simulink model "MotionPlanner"  (R2024b)
settings: Solver=FixedStepAuto  StartTime=0.0  StopTime=10.0  MaxStep=0.02  RelTol=1e-3  EnableMultiTasking=on
undefined symbols (not defined in the file or in its folder): actorProfiles, computeMethod, replanRate, timeResolution, Ts
libraries: simulink x1
settings Model: Creator=The MathWorks, Inc.  LastModifiedBy=The MathWorks, Inc.
settings SolverCC: AlgebraicLoopSolver=TrustRegion  MaxZcPerStep=1
settings OptimizationCC: DefaultParameterBehavior=Inlined  InlineInvariantSignals=on  EnhancedBackFolding=on  PassReuseOutputArgsAs=Individual arguments  ZeroExternalMemoryAtStartup=off  ZeroInternalMemoryAtStartup=off  EfficientFloat2IntCast=on  OptimizeBlockOrder=speed  DifferentSizesBufferReuse=on  OptimizationCustomize=off  EfficientTunableParamExpr=on
settings DebuggingCC: ParameterTunabilityLossMsg=error  UnconnectedInputMsg=warning  UnconnectedOutputMsg=warning  UnconnectedLineMsg=warning  ModelReferenceSymbolNameMessage=none  SubsystemReferenceDiagnosticForUnitTest=warning
settings HardwareCC: ProdLongLongMode=on
settings ModelReferenceCC: EnableRefExpFcnMdlSchedulingChecks=on  PropagateVarSize=During execution
settings RTWCC: Description=Embedded Coder  SystemTargetFile=ert.tlc  TemplateMakefile=ert_default_tmf  RTWVerbose=off  BuildConfiguration=Faster Runs  PortableWordSizes=on  TargetLang=C++  GPUComputeCapability=3.5  DLArmComputeVersion=19.05
settings CodeAppCC: ForceParamTrailComments=on  IgnoreCustomStorageClasses=off  OperatorAnnotations=on  SimulinkDataObjDesc=on  SFDataObjDesc=on  CustomSymbolStrGlobalVar=$N$M  CustomSymbolStrType=$N$M_T  CustomSymbolStrFcn=APV_$N$M$F  CustomSymbolStrMacro=$N$M  InsertBlockDesc=on
settings ERTTargetCC: TargetLangStandard=C++03 (ISO)  GenerateSampleERTMain=on  CombineSignalStateStructs=on  CodeInterfacePackaging=C++ class  SupportVariableSizeSignals=on  RootIOFormat=Structure reference  ERTCustomFileTemplate=example_file_process.tlc  DynamicArrayContainerType=coder::array

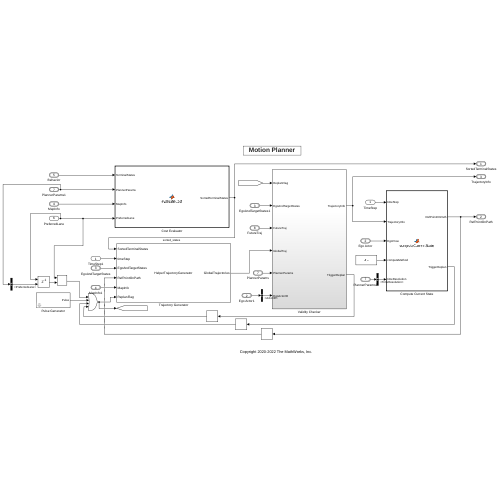
[thumbnail: Simulink's stored preview of the top-level diagram]
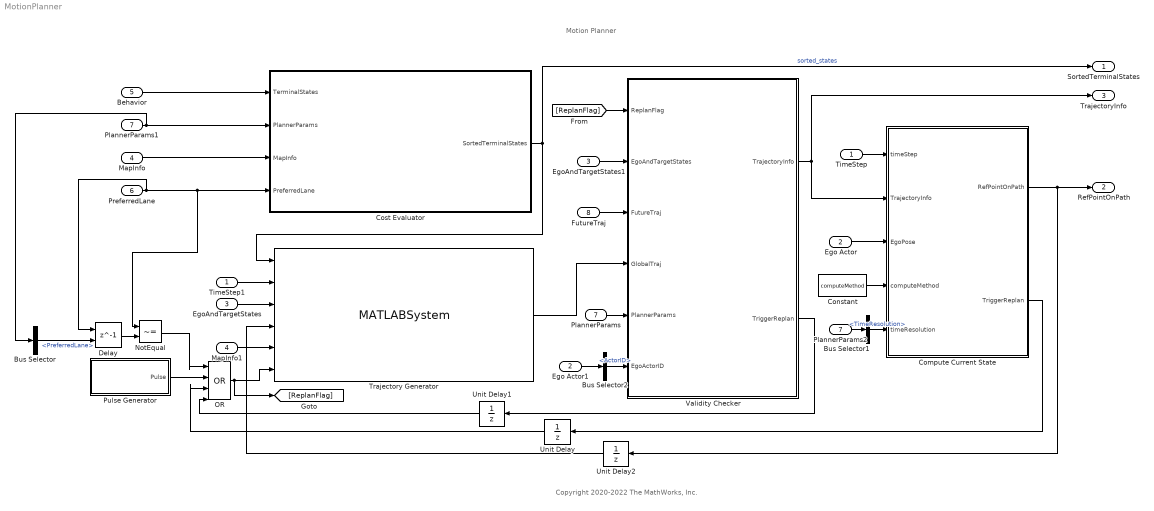
== system MotionPlanner ==
  note: Motion Planner
  note: Copyright 2020-2022 The MathWorks, Inc.
  TimeStep : Inport
  Ego Actor : Inport  Port=2  OutDataTypeStr=Bus: BusVehiclePose  Unit=m  BusOutputAsStruct=on
  EgoAndTargetStates : Inport  Port=3  OutDataTypeStr=Bus: BusEgoAndTargetStates  BusOutputAsStruct=on
  MapInfo : Inport  Port=4  OutDataTypeStr=Bus: BusMapInfo  BusOutputAsStruct=on
  Behavior : Inport  Port=5  OutDataTypeStr=Bus: BusTerminalStatesCombinations
  PreferredLane : Inport  Port=6
  PlannerParams : Inport  Port=7  OutDataTypeStr=Bus: BusPlannerParams  BusOutputAsStruct=on
  FutureTraj : Inport  Port=8  OutDataTypeStr=Bus: BusPredictedTrajectories  BusOutputAsStruct=on
  Bus Selector : BusSelector  OutputSignals=PreferredLane
  Bus Selector1 : BusSelector  OutputSignals=TimeResolution
  Bus Selector2 : BusSelector  OutputSignals=ActorID
  Compute Current State : MATLAB Function  TreatAsAtomicUnit=on
  Constant : Constant  Value=computeMethod
  Cost Evaluator : MATLAB Function  TreatAsAtomicUnit=on
  Delay : Delay  DelayLength=1  InitialConditionSource=Input port
      settings: InputPortMap=u0,p4
  Ego Actor1 : InportShadow  Port=2  OutDataTypeStr=Bus: BusVehiclePose  Unit=m  BusOutputAsStruct=on
  EgoAndTargetStates1 : InportShadow  Port=3  OutDataTypeStr=Bus: BusEgoAndTargetStates  BusOutputAsStruct=on
  MapInfo1 : InportShadow  Port=4  OutDataTypeStr=Bus: BusMapInfo  BusOutputAsStruct=on
  NotEqual : RelationalOperator  Operator=~=  OutDataTypeStr=boolean  RndMeth=Simplest  InputSameDT=off
  OR : Logic  Operator=OR  Inputs=4  IconShape=distinctive  AllPortsSameDT=off  OutDataTypeStr=boolean
  PlannerParams1 : InportShadow  Port=7  OutDataTypeStr=Bus: BusPlannerParams  BusOutputAsStruct=on
  PlannerParams2 : InportShadow  Port=7  OutDataTypeStr=Bus: BusPlannerParams  BusOutputAsStruct=on
  Pulse Generator : Subsystem  mask(Pulse Generator){pulsePeriod=1/replanRate, sampleTime=timeResolution}
      mask prompts: pulsePeriod "Pulse period (sec)"; sampleTime "Sample time (sec)"
      mask help: Generates a periodic pulse. The pulse is high for the first sample of the period and then is low for the remained of the period.
  TimeStep1 : InportShadow
  Trajectory Generator : MATLABSystem  System=HelperTrajectoryGenerator  SimulateUsing=Interpreted execution
      mask Type: HelperTrajectoryGenerator
      mask Display:
      | disp('HelperTrajectoryGenerator');
      | port_label('input',1,'SortedTerminalStates');
      | port_label('input',2,'timeStep');
      | port_label('input',3,'EgoAndTargetStates');
      | port_label('input',4,'RefPointOnPath');
      | port_label('input',5,'MapInfo');
      | port_label('input',6,'ReplanFlag');
      | port_label('output',1,'GlobalTrajectories');
  Unit Delay : UnitDelay  InitialCondition=false  SampleTime=-1  HasFrameUpgradeWarning=on
  Unit Delay1 : UnitDelay  InitialCondition=false  SampleTime=-1  HasFrameUpgradeWarning=on
  Unit Delay2 : UnitDelay  SampleTime=-1  HasFrameUpgradeWarning=on
  Validity Checker : Subsystem
  SortedTerminalStates : Outport  OutDataTypeStr=Bus: BusTerminalStatesCombinations  BusOutputAsStruct=on
  RefPointOnPath : Outport  Port=2  OutDataTypeStr=Bus: BusRefPointOnPath
  TrajectoryInfo : Outport  Port=3  OutDataTypeStr=Bus: BusGlobalTrajectories  BusOutputAsStruct=on
  wires:
  NotEqual/1 -> OR/1
  PlannerParams1/1 -> Bus Selector/1, Cost Evaluator/2(PlannerParams)
  PreferredLane/1 -> NotEqual/1, Cost Evaluator/4(PreferredLane), Delay/1
  Unit Delay1/1 -> OR/4
  Compute Current State/1(RefPointOnPath) -> RefPointOnPath/1, Unit Delay2/1
  Ego Actor/1 -> Compute Current State/3(EgoPose)
  Cost Evaluator/1(SortedTerminalStates) -> SortedTerminalStates/1, Trajectory Generator/1  "sorted_states"
  [ReplanFlag] -> Validity Checker/1(ReplanFlag)
  Ego Actor1/1 -> Bus Selector2/1
  Delay/1 -> NotEqual/2
  MapInfo/1 -> Cost Evaluator/3(MapInfo)
  TimeStep1/1 -> Trajectory Generator/2
  Constant/1 -> Compute Current State/4(computeMethod)
  Bus Selector1/1 -> Compute Current State/5(timeResolution)  "<TimeResolution>"
  TimeStep/1 -> Compute Current State/1(timeStep)
  PlannerParams2/1 -> Bus Selector1/1
  Pulse Generator/1(Pulse) -> OR/2
  Bus Selector2/1 -> Validity Checker/6(EgoActorID)  "<ActorID>"
  Compute Current State/2(TriggerReplan) -> Unit Delay/1
  MapInfo1/1 -> Trajectory Generator/5
  Bus Selector/1 -> Delay/2  "<PreferredLane>"
  Unit Delay2/1 -> Trajectory Generator/4
  OR/1 -> Trajectory Generator/6, [ReplanFlag]
  Unit Delay/1 -> OR/3
  Validity Checker/2(TriggerReplan) -> Unit Delay1/1
  FutureTraj/1 -> Validity Checker/3(FutureTraj)
  Behavior/1 -> Cost Evaluator/1(TerminalStates)
  EgoAndTargetStates/1 -> Trajectory Generator/3
  Validity Checker/1(TrajectoryInfo) -> Compute Current State/2(TrajectoryInfo), TrajectoryInfo/1
  EgoAndTargetStates1/1 -> Validity Checker/2(EgoAndTargetStates)
  PlannerParams/1 -> Validity Checker/5(PlannerParams)
  Trajectory Generator/1 -> Validity Checker/4(GlobalTraj)

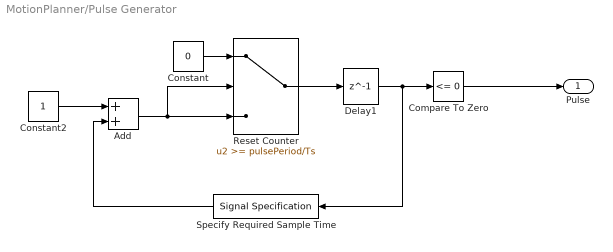
== system MotionPlanner/Pulse Generator ==
  Add : Sum
  Compare To Zero : simulink/Logic and Bit Operations/Compare To Zero  relop=<=  OutDataTypeStr=boolean
  Constant : Constant  Value=0
  Constant2 : Constant
  Delay1 : Delay  DelayLength=1
  Reset Counter : Switch  Threshold=pulsePeriod/Ts  SaturateOnIntegerOverflow=off  InputSameDT=off
      settings: AttributesFormatString=|
      | ----------------------------
      | Threshold = %<Threshold>
  Specify Required Sample Time : SignalSpecification  SampleTime=sampleTime
  Pulse : Outport
  wires:
  Reset Counter/1 -> Delay1/1
  Add/1 -> Reset Counter/3, Reset Counter/2
  Specify Required Sample Time/1 -> Add/2
  Delay1/1 -> Specify Required Sample Time/1, Compare To Zero/1
  Constant2/1 -> Add/1
  Constant/1 -> Reset Counter/1
  Compare To Zero/1 -> Pulse/1

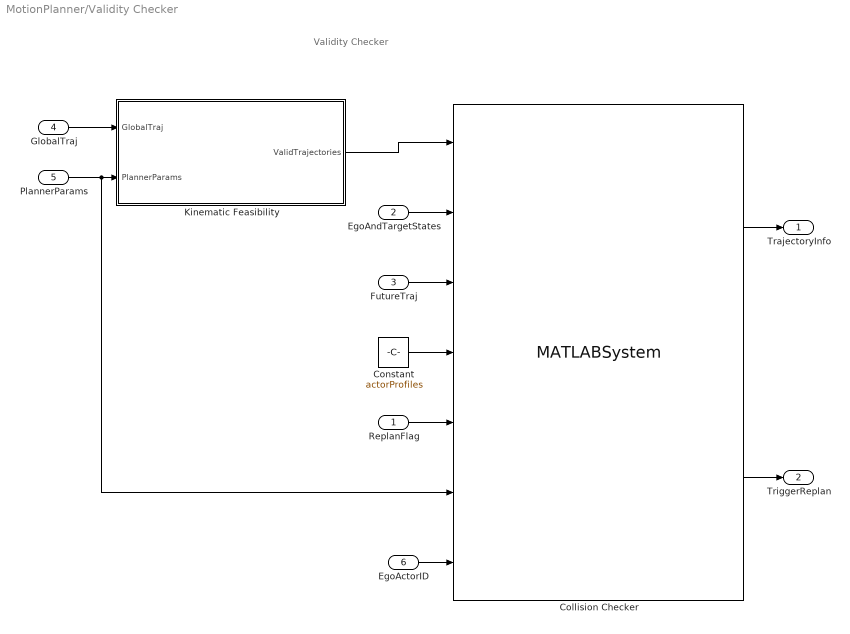
== system MotionPlanner/Validity Checker ==
  note: Validity Checker
  ReplanFlag : Inport
  EgoAndTargetStates : Inport  Port=2
  FutureTraj : Inport  Port=3
  GlobalTraj : Inport  Port=4
  PlannerParams : Inport  Port=5  OutDataTypeStr=Bus: BusPlannerParams
  EgoActorID : Inport  Port=6
  Collision Checker : MATLABSystem  System=HelperCollisionChecker  SimulateUsing=Interpreted execution
      mask Type: HelperCollisionChecker
      mask Display:
      | disp('HelperCollisionChecker');
      | port_label('input',1,'ValidTrajectories');
      | port_label('input',2,'EgoAndTargetStates');
      | port_label('input',3,'FutureTrajectory');
      | port_label('input',4,'VehicleProfiles');
      | port_label('input',5,'ReplanFlag');
      | port_label('input',6,'PlannerParams');
      | port_label('input',7,'EgoID');
      | port_label('output',1,'TrajectoryInfo');
      | port_label('output',2,'TriggerReplan');
  Constant : Constant  Value=actorProfiles  OutDataTypeStr=Bus: BusActorProfiles
  Kinematic Feasibility : MATLAB Function  TreatAsAtomicUnit=on
  TrajectoryInfo : Outport
  TriggerReplan : Outport  Port=2
  wires:
  Collision Checker/1 -> TrajectoryInfo/1
  FutureTraj/1 -> Collision Checker/3
  ReplanFlag/1 -> Collision Checker/5
  Constant/1 -> Collision Checker/4
  Kinematic Feasibility/1(ValidTrajectories) -> Collision Checker/1
  EgoAndTargetStates/1 -> Collision Checker/2
  Collision Checker/2 -> TriggerReplan/1
  GlobalTraj/1 -> Kinematic Feasibility/1(GlobalTraj)
  PlannerParams/1 -> Collision Checker/6, Kinematic Feasibility/2(PlannerParams)
  EgoActorID/1 -> Collision Checker/7

== matlab function MotionPlanner/Compute Current State ==
  data: timeStep input; TrajectoryInfo input; RefPointOnPath output Bus: BusRefPointOnPath; EgoPose input; TriggerReplan output; computeMethod input; timeResolution input
function [RefPointOnPath, TriggerReplan]  = computeCurrentState(timeStep, TrajectoryInfo,...
                                            EgoPose, computeMethod, timeResolution)...
%computeCurrentState estimates the next state of the vehicle based on the
%time or current pose of the ego vehicle.
%
% This function block estimate sthe current pose of the ego vehicle based
% on time or based on current ego pose based on the input from
% StateSelector. If the StateSelector is zero it estimates the pose based
% on current pose, otherwise it estimates state based on time.

persistent replanTime refPosePrev refCurvPrev refVelPrev refAccPrev sectionStartIndexPrev time
if isempty(replanTime)
    replanTime = 0;
    refPosePrev = zeros(1,3);
    refCurvPrev = 0;
    refVelPrev = 0;
    refAccPrev = 0;
    sectionStartIndexPrev = 0;
    time = 0;
end

if TrajectoryInfo.IsNew
    replanTime = time;
end

% Initialize output structure
RefPointOnPath = HelperLCPlannerDefaultData.RefPointOnPath;

optimalTrajIndex = TrajectoryInfo.OptimalTrajectoryIndex;
optimalTrajectory = TrajectoryInfo.GlobalTrajectory(optimalTrajIndex).Trajectory;
numTrajPoints = TrajectoryInfo.GlobalTrajectory(optimalTrajIndex).NumTrajPoints;
times = TrajectoryInfo.GlobalTrajectory(optimalTrajIndex).Times;

% Check StateSelector
if computeMethod == 1
 % Select state based on time
 [RefPoseRr,RefCurvature,...
  RefVelocity,RefAccel,...
  RefAngVel,RefCurvatureDer,...
  LatOffset,RefYawDiff,...
  TriggerReplan] = helperComputeCurrentStateBasedOnTime(time,...
                                                      replanTime,...
                                                      numTrajPoints,...
                                                      optimalTrajectory,...
                                                      times, ...
                                                      timeResolution);                                                  
else
    % Select state based on current pose
   currentPose = [EgoPose.Position(1:2) EgoPose.Yaw];
   [~, refPoses,...
    refCurva, refVelo,...
    refAcc, refAngVel,...
    refCurvDer]  = helperConvertToFixedHorizon(TrajectoryInfo.IsNew,...
                                               numTrajPoints,...
                                               optimalTrajectory, times);

  [~,...
   RefPoseRr,...
   RefCurvature,...
   RefVelocity,...
   RefAccel,...
   RefAngVel, RefCurvatureDer,...
   LatOffset,RefYawDiff,...
   sectionStartIndex] = helperComputeCurrentStateBasedOnPose(currentPose,...
                                                          TrajectoryInfo.IsNew,...
                                                          refPoses,...
                                                          refCurva, refVelo,...
                                                          refAcc, refAngVel,...
                                                          refCurvDer,...
                                                          refPosePrev,...
                                                          refCurvPrev,...
                                                          refVelPrev,...
                                                          refAccPrev,...
                                                          sectionStartIndexPrev);
    
    if sectionStartIndex > numTrajPoints
        TriggerReplan = true;
    else
        TriggerReplan = false;
    end
    refPosePrev = RefPoseRr;
    refCurvPrev = RefCurvature;
    refVelPrev = RefVelocity;
    refAccPrev = RefAccel;
    sectionStartIndexPrev = sectionStartIndex;                                                 
end

RefPointOnPath.CurrPoseRr       = [EgoPose.Position(1:2) EgoPose.Yaw];
RefPointOnPath.RefPoseRr        = RefPoseRr;
RefPointOnPath.LatOffset        = LatOffset;
RefPointOnPath.RefCurvature     = RefCurvature;
RefPointOnPath.RefCurvatureDer  = RefCurvatureDer;
RefPointOnPath.RefYawDiff       = RefYawDiff;
RefPointOnPath.RefVelocity      = RefVelocity;
RefPointOnPath.RefAccel         = RefAccel;
RefPointOnPath.RefAngVel        = RefAngVel;

time = time + timeStep;
end

== matlab function MotionPlanner/Cost Evaluator ==
  data: TerminalStates input; PlannerParams input; MapInfo input; SortedTerminalStates output Bus: BusTerminalStatesCombinations; PreferredLane input
function SortedTerminalStates = evaluateCost(TerminalStates,...
                                                    PlannerParams,...
                                                    MapInfo,...
                                                    PreferredLane)
%evaluateCost function block evaluates the terminal states using the
%weights specified and sorth the terminal states in ascending order of
%weights.
SortedTerminalStates = helperEvaluateCost(TerminalStates,...
                                          PlannerParams,...
                                          MapInfo,...
                                          PlannerParams.SetSpeed,...
                                          PreferredLane);
end

== matlab function MotionPlanner/Validity Checker/Kinematic Feasibility ==
  data: GlobalTraj input; ValidTrajectories output Bus: BusGlobalTrajectories; PlannerParams input
function ValidTrajectories = checkKinematicFeasibility(GlobalTraj,...
                                                       PlannerParams)
%checkKinematicFeasibility checks for kinematic feasibility of generated
%global trjaectories. It invokes helperKinematicFeasibility for calculating
%the feasibility and update the GlobalTraj struct.
ValidTrajectories = helperKinematicFeasibility(GlobalTraj, PlannerParams);
end
